simulink library "powerlib_modelsV2"  (Simulink 6.0)
settings: Solver=ode45  SolverMode=SingleTasking  StartTime=0.0  StopTime=10.0  RelTol=1e-3
undefined symbols (not defined in the file or in its folder): A, Ac, B, Bc, C, Cc, Cs, Current, damp, Dc, Dd, DiscIntNeverNeededParam, dref, dwo, exc, F, fb, gate, GH, GHd, GI, GId, GL, GLd, H, HT, hyd, ib, ib2, io, isfinite, j, K, Kd, Kg, L, Lad, Laq, lim, LIM, Ll, Llfd, Llkd, Llkq1, Llkq2, Llr, Lls, LowerFlux, N, N2, Nb, Nb2, nb_arm, p, Par_HarmoA_pu, Par_HarmoB_pu, Par_Timing_Harmo, Par_Timing_Variation, Par_Vps, Pb ... (+58)
libraries: powerlib_extras x14
(part 6 of 11)

== system powerlib_modelsV2/Continuous/Dynamic_Load/Break  Alg. Loop ==
  In : Inport  Orientation=left  Port=1  LatchInput=off
  Complex to Real-Imag : ComplexToRealImag  Orientation=left
  Real-Imag to Complex : RealImagToComplex  Orientation=left
  imag : Subsystem  Orientation=left  AncestorBlock=|  mask(Transfer Function with Initial Outputs){N=[1], D=[100e-6  1], Y0=imag(I1_init*exp(-j*Pha_V0*pi/180)), U0=imag(I1_init*exp(-j*Pha_V0*pi/180))}
      | simulink_extras/Additional
      | Linear/Transfer Fcn
      | (with initial outputs)
      mask prompts: N "Numerator:"; D "Denominator:"; Y0 "Initial output:"; U0 "Initial input:"
      mask help: Vector expressions for numerator, and denominator. Coefficients are in descending powers of s.
      mask init:
      | [A,B,C,Dd]=tf2ss(N,D);if (isempty(Y0));[m,n]=size(A);X0=zeros(1,m); end; if (isempty(U0));[m,p]=size(B);U0=zeros(1,p);end;X0=getxo(A,B,C,Dd,U0,Y0,0);
      mask Help: Specify the initial output for the transfer function.  An optimization routine attempts to determine the appropriate initial states so that the specified initial output is achieved.  For more details, see the m-file getxo.m
      mask Display: dpoly(N,D,'s')
  real : Subsystem  Orientation=left  AncestorBlock=|  mask(Transfer Function with Initial Outputs){N=[1], D=[100e-6  1], Y0=real(I1_init*exp(-j*Pha_V0*pi/180)), U0=real(I1_init*exp(-j*Pha_V0*pi/180))}
      | simulink_extras/Additional
      | Linear/Transfer Fcn
      | (with initial outputs)
      mask prompts: N "Numerator:"; D "Denominator:"; Y0 "Initial output:"; U0 "Initial input:"
      mask help: Vector expressions for numerator, and denominator. Coefficients are in descending powers of s.
      mask init:
      | [A,B,C,Dd]=tf2ss(N,D);if (isempty(Y0));[m,n]=size(A);X0=zeros(1,m); end; if (isempty(U0));[m,p]=size(B);U0=zeros(1,p);end;X0=getxo(A,B,C,Dd,U0,Y0,0);
      mask Help: Specify the initial output for the transfer function.  An optimization routine attempts to determine the appropriate initial states so that the specified initial output is achieved.  For more details, see the m-file getxo.m
      mask Display: dpoly(N,D,'s')
  Out : Outport  Orientation=left
  wires:
  In/1 -> Complex to Real-Imag/1
  Real-Imag to Complex/1 -> Out/1
  Complex to Real-Imag/1 -> real/1(In1)
  real/1(Out1) -> Real-Imag to Complex/1
  Complex to Real-Imag/2 -> imag/1(In1)
  imag/1(Out1) -> Real-Imag to Complex/2

== system powerlib_modelsV2/Continuous/Dynamic_Load/Positive Sequence  current ==
  note: I1= (S/V1)'
  note: V>Vmin :
      |
      |    P=Po*(V/Vo)^np
      |    Q=Qo*(V/Vo)^np
  note: V<Vmin
      | Constant impedance load :
      |
      |  P=Po*kp*V^2
      | Q=Qo*kq*V^2
  note: kp=Vmin^(np-2)/Vo^np
      | kq=Vmin^(nq-2)/Vo^nq
  V1(pu) : Inport  Port=1  LatchInput=off
  S_ext : Inport  Port=2  LatchInput=off
  Complex to Magnitude-Angle : ComplexToMagnitudeAngle  Output=Magnitude
  Complex to Real-Imag1 : ComplexToRealImag
  Conj1 : Math  Operator=conj  SaturateOnIntegerOverflow=on
  Math Function : Math  Operator=square  SaturateOnIntegerOverflow=on
  Mux1 : Mux  Inputs=3
  Mux2 : Mux  Inputs=2
  Mux3 : Mux  Inputs=2
  P0/ (Vo^np) : Gain  Gain=P0/(Mag_V0^np)  SaturateOnIntegerOverflow=on
  PQ_ext : Constant  Value=PQext
  Product : Product  Inputs=/*  SaturateOnIntegerOverflow=on  InputSameDT=on
  Q0/(Vo^nq) : Gain  Gain=Q0/(Mag_V0^nq)  SaturateOnIntegerOverflow=on
  Real-Imag to Complex : RealImagToComplex
  Switch1 : Switch  Threshold=0.5  InputSameDT=on
  Switch3 : Switch  Threshold=Vmin  InputSameDT=on
  Switch4 : Switch  Threshold=Vmin  InputSameDT=on
  TF_P : Subsystem  mask(Transfer function){T1=Tp1, T2=Tp2, V_Init=P0}
      mask prompts: T1 "Time constant T1 (s):"; T2 "Time constant T2 (s):"; V_Init "Initial input and output :"
      mask help:
      | This block implements a continuous transfer function:
      |
      |          1+T1s
      | H(s)= ------
      |          1+T2s
      |
      | States are initialized according to  initial input and output value so that simulation starts in steady state.
      mask init:
      | numc=[T1 1];
      | denc=[T2 1];
      | [Ac,Bc,Cc,Dc]=tf2ss(numc,denc);
      | 
      | % Compute Initial states
      | I=eye(size(Ac));
      | x0c=inv(-Ac)*Bc*V_Init;
      mask Display: disp('1+T1s\n---\n1+T2s')
  TF_Q : Subsystem  mask(Transfer function){T1=Tq1, T2=Tq2, V_Init=Q0}
      mask prompts: T1 "Time constant T1 (s):"; T2 "Time constant T2 (s):"; V_Init "Initial input and output :"
      mask help:
      | This block implements a continuous transfer function:
      |
      |          1+T1s
      | H(s)= ------
      |          1+T2s
      |
      | States are initialized according to  initial input and output value so that simulation starts in steady state.
      mask init:
      | numc=[T1 1];
      | denc=[T2 1];
      | [Ac,Bc,Cc,Dc]=tf2ss(numc,denc);
      | 
      | % Compute Initial states
      | I=eye(size(Ac));
      | x0c=inv(-Ac)*Bc*V_Init;
      mask Display: disp('1+T1s\n---\n1+T2s')
  V^nq : Fcn  Expr=u[1]^u[2]
  V^nq , : Fcn  Expr=u[1]^u[2]
  Vmin^(np-2) : Gain  Gain=Vmin^(np-2)  SaturateOnIntegerOverflow=on
  Vmin^(nq-2) : Gain  Gain=Vmin^(nq-2)  SaturateOnIntegerOverflow=on
  np : Constant  Value=np
  nq : Constant  Value=nq
  pu>V : Gain  Gain=Vnom*sqrt(3)/sqrt(2)  SaturateOnIntegerOverflow=on
  I1(A) : Outport
  VPQ : Outport  Port=2
  wires:
  TF_Q/1(Out1) -> Real-Imag to Complex/2
  TF_P/1(Out1) -> Real-Imag to Complex/1
  Complex to Real-Imag1/2 -> Mux1/3
  Complex to Real-Imag1/1 -> Mux1/2
  Mux1/1 -> VPQ/1
  Complex to Magnitude-Angle/1 -> Mux1/1, Switch4/2, Switch3/2, Mux2/1, Mux3/1, Math Function/1
  pu>V/1 -> Product/1
  PQ_ext/1 -> Switch1/2
  S_ext/1 -> Switch1/1
  Real-Imag to Complex/1 -> Switch1/3  "S_dyn"
  Switch1/1 -> Complex to Real-Imag1/1, Product/2  "S=P+jQ"
  Conj1/1 -> I1(A)/1
  Product/1 -> Conj1/1
  Switch4/1 -> Q0/(Vo^nq)/1
  P0/ (Vo^np)/1 -> TF_P/1(In1)
  Q0/(Vo^nq)/1 -> TF_Q/1(In1)
  Switch3/1 -> P0/ (Vo^np)/1
  np/1 -> Mux2/2
  Mux2/1 -> V^nq ,/1
  nq/1 -> Mux3/2
  Mux3/1 -> V^nq/1
  V1(pu)/1 -> pu>V/1, Complex to Magnitude-Angle/1
  V^nq/1 -> Switch4/1
  Math Function/1 -> Vmin^(np-2)/1, Vmin^(nq-2)/1
  Vmin^(np-2)/1 -> Switch3/3
  V^nq ,/1 -> Switch3/1
  Vmin^(nq-2)/1 -> Switch4/3

== system powerlib_modelsV2/Continuous/Dynamic_Load/Variable Frequency Mean value1 ==
  note: Pierre Giroux, Gilbert Sybille
      | Power System Simulation Laboratory
      | IREQ, Hydro-Quebc
  note: Mean Value (Variable frequency)
  Freq : Inport  Port=1  LatchInput=off
  In : Inport  Port=2  LatchInput=off
  Constant : Constant  Value=Vinit
  Integrator : Integrator
  Number of samples per cycle : Fcn  Expr=1/u[1]
  Product : Product  SaturateOnIntegerOverflow=on  InputSameDT=on
  Step : Step  Time=1/Finit  SampleTime=0
  Sum7 : Sum  Inputs=-+  SaturateOnIntegerOverflow=on  InputSameDT=on
  Switch : Switch  Threshold=0.5  InputSameDT=on
  To avoid division by zero : Saturate  Orientation=down  UpperLimit=1e6  LowerLimit=1e-6
  Variable Transport Delay : VariableTransportDelay  MaximumDelay=1/40  MaximumPoints=4096
  Mean : Outport
  wires:
  In/1 -> Integrator/1  "In"
  Product/1 -> Switch/1  "Mean value"
  Variable Transport Delay/1 -> Sum7/1
  Sum7/1 -> Product/1
  Integrator/1 -> Sum7/2, Variable Transport Delay/1
  Freq/1 -> Product/2, To avoid division by zero/1  "Freq"
  Constant/1 -> Switch/3
  Switch/1 -> Mean/1
  To avoid division by zero/1 -> Number of samples per cycle/1  "Freq"
  Step/1 -> Switch/2
  Number of samples per cycle/1 -> Variable Transport Delay/2  "Delay"

== system powerlib_modelsV2/Continuous/Dynamic_Load/Variable Frequency Mean value2 ==
  note: Mean Value (Variable frequency)
  note: Pierre Giroux, Gilbert Sybille
      | Power System Simulation Laboratory
      | IREQ, Hydro-Quebc
  Freq : Inport  Port=1  LatchInput=off
  In : Inport  Port=2  LatchInput=off
  Constant : Constant  Value=Vinit
  Integrator : Integrator
  Number of samples per cycle : Fcn  Expr=1/u[1]
  Product : Product  SaturateOnIntegerOverflow=on  InputSameDT=on
  Step : Step  Time=1/Finit  SampleTime=0
  Sum7 : Sum  Inputs=-+  SaturateOnIntegerOverflow=on  InputSameDT=on
  Switch : Switch  Threshold=0.5  InputSameDT=on
  To avoid division by zero : Saturate  Orientation=down  UpperLimit=1e6  LowerLimit=1e-6
  Variable Transport Delay : VariableTransportDelay  MaximumDelay=1/40  MaximumPoints=4096
  Mean : Outport
  wires:
  Number of samples per cycle/1 -> Variable Transport Delay/2  "Delay"
  Step/1 -> Switch/2
  To avoid division by zero/1 -> Number of samples per cycle/1  "Freq"
  Switch/1 -> Mean/1
  Constant/1 -> Switch/3
  Freq/1 -> To avoid division by zero/1, Product/2  "Freq"
  Integrator/1 -> Variable Transport Delay/1, Sum7/2
  Sum7/1 -> Product/1
  Variable Transport Delay/1 -> Sum7/1
  Product/1 -> Switch/1  "Mean value"
  In/1 -> Integrator/1  "In"

== system powerlib_modelsV2/Continuous/Dynamic_Load/dq0_to_abc Transformation ==
  note: Va= Vd*sinwt + Vq*cos(wt) + Vo
  note: sin
  note: cos
  note: cos
  note: Vb= Vd*sin(wt-2pi/3) + Vq*cos(wt-2pi/3) + Vo
  note: Vc= Vd*sin(wt+2pi/3) + Vq*cos(wt+2pi/3) + Vo
  dq0 : Inport  Port=1  PortDimensions=3  LatchInput=off
  sin_cos : Inport  Port=2  PortDimensions=2  LatchInput=off
  Demux : Demux  Outputs=2
  Fcn2 : Fcn  Expr="u[1]*u[4] +  u[2]*u[5] + u[3]"
  Fcn4 : Fcn  Expr="u[1]*u[6] +  u[2]*u[7]+ u[3]"
  Fcn5 : Fcn  Expr="u[1]*u[8]+  u[2]*u[9]+ u[3]"
  K1 : Constant  Value=0.5
  K2 : Constant  Value=sqrt(3)/2
  Mux : Mux  Inputs=2
  Mux1 : Mux  Inputs=3
  Mux2 : Mux  Inputs=6
  Product{,1..3} (4 alike) : Product  SaturateOnIntegerOverflow=on  InputSameDT=on
  Sum : Sum  Inputs=--  SaturateOnIntegerOverflow=on  InputSameDT=on
  Sum1 : Sum  Inputs=-+  SaturateOnIntegerOverflow=on  InputSameDT=on
  Sum2 : Sum  Inputs=--  SaturateOnIntegerOverflow=on  InputSameDT=on
  Sum3 : Sum  Inputs=--  SaturateOnIntegerOverflow=on  InputSameDT=on
  abc : Outport  InitialOutput=0
  wires:
  Fcn5/1 -> Mux1/3  "Vc"
  Fcn2/1 -> Mux1/1  "Va"
  Mux1/1 -> abc/1
  Mux/1 -> Fcn4/1, Fcn2/1, Fcn5/1
  Sum1/1 -> Sum3/1, Mux2/4  "cos(wt-2pi/3)"
  Sum/1 -> Sum2/1, Mux2/3  "sin(wt-2pi/3)"
  K2/1 -> Product2/2, Product1/2
  K1/1 -> Product3/2, Product/2
  Sum2/1 -> Mux2/5  "sin(wt+2pi/3)"
  Sum3/1 -> Mux2/6  "cos(wt+2pi/3)"
  Product2/1 -> Sum1/2
  Product3/1 -> Sum1/1
  Product1/1 -> Sum/2
  Product/1 -> Sum/1
  Demux/1 -> Mux2/1, Sum2/2, Product2/1, Product/1  "sin(wt)"
  Demux/2 -> Mux2/2, Product1/1, Product3/1, Sum3/2  "cos(wt)"
  sin_cos/1 -> Demux/1
  Mux2/1 -> Mux/2
  dq0/1 -> Mux/1  "Vabc"
  Fcn4/1 -> Mux1/2  "Vb"

== system powerlib_modelsV2/Continuous/Excitation_System/Damping kf.s\ (tf.s +1) ==
  In1 : Inport  Port=1  LatchInput=off
  State Space : StateSpace  A=A  B=B  C=C  D=Dd  X0=X0
  Out1 : Outport  InitialOutput=0
  wires:
  State Space/1 -> Out1/1
  In1/1 -> State Space/1

== system powerlib_modelsV2/Continuous/Excitation_System/Exciter 1 \(te.s +ke) ==
  In1 : Inport  Port=1  LatchInput=off
  State Space : StateSpace  A=A  B=B  C=C  D=Dd  X0=X0
  Out1 : Outport  InitialOutput=0
  wires:
  In1/1 -> State Space/1
  State Space/1 -> Out1/1

== system powerlib_modelsV2/Continuous/Excitation_System/Lead Lag Compensator tc.s+1\tb.s+1 ==
  In1 : Inport  Port=1  LatchInput=off
  State Space : StateSpace  A=A  B=B  C=C  D=Dd  X0=X0
  Out1 : Outport  InitialOutput=0
  wires:
  State Space/1 -> Out1/1
  In1/1 -> State Space/1

== system powerlib_modelsV2/Continuous/Excitation_System/Low Pass Filter 1 \ (tr.s+1) (with IC) ==
  In1 : Inport  Port=1  LatchInput=off
  State Space : StateSpace  A=A  B=B  C=C  D=Dd  X0=X0
  Out1 : Outport  InitialOutput=0
  wires:
  In1/1 -> State Space/1
  State Space/1 -> Out1/1

== system powerlib_modelsV2/Continuous/Excitation_System/Main Regulator ka \ (ta.s+1) ==
  In1 : Inport  Port=1  LatchInput=off
  State Space : StateSpace  A=A  B=B  C=C  D=Dd  X0=X0
  Out1 : Outport  InitialOutput=0
  wires:
  State Space/1 -> Out1/1
  In1/1 -> State Space/1

== system powerlib_modelsV2/Continuous/Excitation_System/proportionnal saturation ==
  Efd : Inport  Port=1  LatchInput=off
  Vtf : Inport  Port=2  LatchInput=off
  Constant : Constant  Value=kp
  Constant1 : Constant  Value=efmin
  Constant3 : Constant  Value=0
  Data Type  Conversion{,1..3} (4 alike) : DataTypeConversion  SaturateOnIntegerOverflow=on  RndMeth=Zero
  Logical Operator : Logic
  Logical Operator1 : Logic  Operator=NOT  Inputs=1
  Logical Operator2 : Logic  Operator=NOT  Inputs=1
  Product : Product  SaturateOnIntegerOverflow=on  InputSameDT=on
  Product1 : Product  SaturateOnIntegerOverflow=on  InputSameDT=on
  Product2 : Product  SaturateOnIntegerOverflow=on  InputSameDT=on
  Relational Operator : RelationalOperator  Operator===  InputSameDT=on
  Relational Operator1 : RelationalOperator  Operator=<  InputSameDT=on
  Relational Operator2 : RelationalOperator  Operator=>  InputSameDT=on
  Sum : Sum  SaturateOnIntegerOverflow=on  InputSameDT=on
  Sum1 : Sum  Inputs=+++  SaturateOnIntegerOverflow=on  InputSameDT=on
  Vfdmax : Gain  Gain=efmax  SaturateOnIntegerOverflow=on
  Vfdmax1 : Gain  Gain=kp  SaturateOnIntegerOverflow=on
  Ef : Outport  InitialOutput=0
  wires:
  Data Type  Conversion3/1 -> Vfdmax/1
  Relational Operator/1 -> Data Type  Conversion3/1
  Data Type  Conversion2/1 -> Product2/1
  Logical Operator2/1 -> Data Type  Conversion2/1
  Data Type  Conversion1/1 -> Product1/2
  Logical Operator1/1 -> Data Type  Conversion1/1
  Data Type  Conversion/1 -> Product/2
  Logical Operator/1 -> Data Type  Conversion/1
  Product1/1 -> Sum1/2
  Product2/1 -> Sum1/3
  Product/1 -> Sum1/1
  Sum1/1 -> Ef/1
  Efd/1 -> Product/1, Relational Operator1/1, Relational Operator2/1
  Constant1/1 -> Product1/1, Relational Operator2/2
  Relational Operator1/1 -> Logical Operator/2, Logical Operator2/1
  Relational Operator2/1 -> Logical Operator/1, Logical Operator1/1
  Sum/1 -> Relational Operator1/2, Product2/2
  Vfdmax1/1 -> Sum/1
  Vfdmax/1 -> Sum/2
  Constant3/1 -> Relational Operator/2
  Constant/1 -> Relational Operator/1
  Vtf/1 -> Vfdmax1/1

== system powerlib_modelsV2/Continuous/GTO-IGBT Bridge/Diode Logic ==
  note: Note : Block D1 (D2) if D2 (D1) is triggered (no Cs)
  Vak : Inport  Port=1  LatchInput=off
  Ipos : Inport  Port=2  LatchInput=off
  G : Inport  Port=3  LatchInput=off
  0 2 : Constant  Value=0
  0 3 : Constant  Value=Cs==inf
  1 : Logic
  2 : Logic  Operator=OR
  3 : Logic  Operator=OR
  Block D : Selector  Orientation=up  Elements=Selec_Diode  InputPortWidth=nb_switch
  Blocking Diodes : Subsystem
  Data Type  Conversion3 : DataTypeConversion  SaturateOnIntegerOverflow=on  RndMeth=Zero
  Logical Operator3 : Logic  Operator=NOT
  Trig.  Diodes (No Snubber Capacitance) : Subsystem  TreatAsAtomicUnit=on
  b6 : RelationalOperator  Operator=>  InputSameDT=on
  status : Outport  InitialOutput=0
  wires:
  0 3/1 -> Trig.  Diodes (No Snubber Capacitance)/Enable
  Ipos/1 -> Trig.  Diodes (No Snubber Capacitance)/2(Ipos)
  G/1 -> Trig.  Diodes (No Snubber Capacitance)/1(G), Blocking Diodes/1(G)
  0 2/1 -> b6/2
  Vak/1 -> b6/1
  Blocking Diodes/1(Block.D) -> 3/1
  2/1 -> status/1
  1/1 -> 2/1
  Logical Operator3/1 -> 1/2
  3/1 -> Logical Operator3/1
  Trig.  Diodes (No Snubber Capacitance)/1(Trig D) -> 2/2, Block D/1
  Block D/1 -> 3/2
  b6/1 -> Data Type  Conversion3/1
  Data Type  Conversion3/1 -> 1/1

== system powerlib_modelsV2/Continuous/GTO-IGBT Bridge/GTO Logic ==
  Vak : Inport  Port=1  LatchInput=off
  G : Inport  Port=2  LatchInput=off
  " " : RelationalOperator  Operator=>  InputSameDT=on
  "    " : Constant  Value=0
  ". " : Logic
  Data Type  Conversion1 : DataTypeConversion  SaturateOnIntegerOverflow=on  RndMeth=Zero
  Data Type  Conversion3 : DataTypeConversion  SaturateOnIntegerOverflow=on  RndMeth=Zero
  Data Type  Conversion4 : DataTypeConversion  SaturateOnIntegerOverflow=on  RndMeth=Zero
  Vpos : Constant  Value=0
  b : RelationalOperator  Operator=>  InputSameDT=on
  status : Outport  InitialOutput=0
  wires:
  ". "/1 -> status/1
  Vak/1 -> b/1
  Vpos/1 -> b/2
  G/1 -> " "/1
  b/1 -> Data Type  Conversion1/1
  Data Type  Conversion1/1 -> ". "/1
  " "/1 -> Data Type  Conversion3/1
  Data Type  Conversion3/1 -> ". "/2
  "    "/1 -> Data Type  Conversion4/1
  Data Type  Conversion4/1 -> " "/2

== system powerlib_modelsV2/Continuous/GTO-IGBT Bridge/Tail  ==
  Iak : Inport  Port=1  LatchInput=off
  switch : Inport  Port=2  LatchInput=off
  Enable : EnablePort  StatesWhenEnabling=reset
  1 : Constant
  2 : Constant  Value=(Tf+Tt)>0
  Data Type  Conversion1 : DataTypeConversion  SaturateOnIntegerOverflow=on  RndMeth=Zero
  Integrator : Integrator  ExternalReset=falling
  Look-Up Table : Lookup  DialogController=Simulink.DDGSource  InputValues="[  0   Tf+eps Tf+Tt+2*eps  Tf+Tt+3*eps]"  OutputValues="[  1   0.1*(Tt>0) 0 0]"  SaturateOnIntegerOverflow=on
  Memory : Memory  Orientation=left  InheritSampleTime=on
  Product : Product  Inputs=3  SaturateOnIntegerOverflow=on  InputSameDT=on
  Switch : Switch  Threshold=0.5  InputSameDT=on
  itail : Outport  InitialOutput=0
  wires:
  2/1 -> Data Type  Conversion1/1
  Look-Up Table/1 -> Product/1
  1/1 -> Integrator/1
  Iak/1 -> Switch/1
  switch/1 -> Switch/2, Integrator/2
  Integrator/1 -> Look-Up Table/1
  Product/1 -> itail/1
  Switch/1 -> Product/2, Memory/1
  Memory/1 -> Switch/3
  Data Type  Conversion1/1 -> Product/3

== system powerlib_modelsV2/Continuous/GTO-IGBT Bridge/Vf  ==
  status_GTO : Inport  Port=1  LatchInput=off
  Switch : Switch  Threshold=0.5  InputSameDT=on
  Vf device : Constant  Value=Vf*ones(nb_switch,1)
  Vf diode : Constant  Value=-Vfd*ones(nb_switch,1)
  Vf : Outport  InitialOutput=[0]
  wires:
  status_GTO/1 -> Switch/2
  Switch/1 -> Vf/1
  Vf diode/1 -> Switch/3
  Vf device/1 -> Switch/1

== system powerlib_modelsV2/Continuous/HTG/PID ==
  error : Inport  Port=1  LatchInput=off
  Derivative : TransferFcn  Numerator=[ kd 0]  Denominator=[ td 1 ]
  Integral : Gain  Gain=ki  SaturateOnIntegerOverflow=on
  Integrator1 : Integrator  InitialCondition=go
  Proportional : Gain  Gain=kp  SaturateOnIntegerOverflow=on
  Sum : Sum  Inputs=+++  SaturateOnIntegerOverflow=on  InputSameDT=on
  Output : Outport  InitialOutput=0
  wires:
  Integrator1/1 -> Sum/2
  Integral/1 -> Integrator1/1
  error/1 -> Integral/1, Proportional/1, Derivative/1
  Sum/1 -> Output/1
  Derivative/1 -> Sum/3
  Proportional/1 -> Sum/1

== system powerlib_modelsV2/Continuous/HTG/servo-motor ==
  regulator's output : Inport  Port=1  LatchInput=off
  Sum4 : Sum  Inputs=+-  SaturateOnIntegerOverflow=on  InputSameDT=on
  position : Integrator  InitialCondition=go  LimitOutput=on  UpperSaturationLimit=gmax  LowerSaturationLimit=gmin
  servo- motor : TransferFcn  Numerator=[ka]  Denominator=[ta 1]
  speed limit : Saturate  UpperLimit=vgmax  LowerLimit=vgmin
  gate opening : Outport  InitialOutput=0
  wires:
  position/1 -> Sum4/2, gate opening/1
  speed limit/1 -> position/1
  servo- motor/1 -> speed limit/1
  Sum4/1 -> servo- motor/1
  regulator's output/1 -> Sum4/1

== system powerlib_modelsV2/Continuous/HTG/turbine ==
  dw : Inport  Port=1  LatchInput=off
  gate opening : Inport  Port=2  LatchInput=off
  Constant : Constant  Orientation=left
  Fcn : Fcn  Expr=(u(2)/u(1))^2
  Gain2 : Gain  Orientation=left  Gain=1/tw  SaturateOnIntegerOverflow=on
  Integrator : Integrator  Orientation=left  InitialCondition=po
  Mux : Mux  Inputs=2
  Product : Product  SaturateOnIntegerOverflow=on  InputSameDT=on
  Sum2 : Sum  Inputs=-+  SaturateOnIntegerOverflow=on  InputSameDT=on
  Sum3 : Sum  Orientation=left  Inputs=-+  SaturateOnIntegerOverflow=on  InputSameDT=on
  beta : Gain  Gain=beta  SaturateOnIntegerOverflow=on
  turbine gain : Gain  Gain=1/(gmax-gmin)  SaturateOnIntegerOverflow=on
  Pm : Outport  InitialOutput=0
  wires:
  turbine gain/1 -> Mux/1
  gate opening/1 -> turbine gain/1
  Integrator/1 -> Product/2, Mux/2
  Mux/1 -> Fcn/1
  Fcn/1 -> Sum2/2
  Constant/1 -> Sum3/2
  Product/1 -> Pm/1
  Sum3/1 -> Gain2/1
  Gain2/1 -> Integrator/1
  Sum2/1 -> Sum3/1, Product/1
  beta/1 -> Sum2/1
  dw/1 -> beta/1

== system powerlib_modelsV2/Continuous/MBPSS/Transfer function for detailed model (HF) ==
  On : Inport  Port=1  LatchInput=off
  "HFpos " : Inport  Port=2  LatchInput=off
  "HFneg " : Inport  Port=3  LatchInput=off
  Switch1 : Switch  Threshold=0.5  InputSameDT=on
  Switch2 : Switch  Threshold=0.5  InputSameDT=on
  Transfer functions for detailed stabilizer : Subsystem  TreatAsAtomicUnit=on
  Transfer functions for detailed stabilizer2 : Subsystem  TreatAsAtomicUnit=on
  HFpos : Outport
  HFneg : Outport  Port=2
  wires:
  Transfer functions for detailed stabilizer/1(Out1) -> Switch1/1
  "HFpos "/1 -> Transfer functions for detailed stabilizer/1(In1), Switch1/3
  Switch1/1 -> HFpos/1
  "HFneg "/1 -> Transfer functions for detailed stabilizer2/1(In1), Switch2/3
  Switch2/1 -> HFneg/1
  Transfer functions for detailed stabilizer2/1(Out1) -> Switch2/1
  On/1 -> Transfer functions for detailed stabilizer/Enable, Switch1/2, Switch2/2, Transfer functions for detailed stabilizer2/Enable

== system powerlib_modelsV2/Continuous/MBPSS/Transfer function for detailed model (IF) ==
  On : Inport  Port=1  LatchInput=off
  "IFpos " : Inport  Port=2  LatchInput=off
  "IFneg " : Inport  Port=3  LatchInput=off
  Switch1 : Switch  Threshold=0.5  InputSameDT=on
  Switch2 : Switch  Threshold=0.5  InputSameDT=on
  Transfer functions for detailed stabilizer : Subsystem  TreatAsAtomicUnit=on
  Transfer functions for detailed stabilizer2 : Subsystem  TreatAsAtomicUnit=on
  IFpos : Outport
  LFneg : Outport  Port=2
  wires:
  On/1 -> Transfer functions for detailed stabilizer2/Enable, Switch2/2, Switch1/2, Transfer functions for detailed stabilizer/Enable
  Transfer functions for detailed stabilizer2/1(Out1) -> Switch2/1
  Switch2/1 -> LFneg/1
  "IFneg "/1 -> Switch2/3, Transfer functions for detailed stabilizer2/1(In1)
  Switch1/1 -> IFpos/1
  "IFpos "/1 -> Switch1/3, Transfer functions for detailed stabilizer/1(In1)
  Transfer functions for detailed stabilizer/1(Out1) -> Switch1/1

== system powerlib_modelsV2/Continuous/MBPSS/Transfer function for detailed model (LF) ==
  On : Inport  Port=1  LatchInput=off
  "LFpos " : Inport  Port=2  LatchInput=off
  "LFneg " : Inport  Port=3  LatchInput=off
  Switch1 : Switch  Threshold=0.5  InputSameDT=on
  Switch2 : Switch  Threshold=0.5  InputSameDT=on
  Transfer functions for detailed stabilizer : Subsystem  TreatAsAtomicUnit=on
  Transfer functions for detailed stabilizer2 : Subsystem  TreatAsAtomicUnit=on
  LFpos : Outport
  LFneg : Outport  Port=2
  wires:
  Transfer functions for detailed stabilizer/1(Out1) -> Switch1/1
  "LFpos "/1 -> Transfer functions for detailed stabilizer/1(In1), Switch1/3
  Switch1/1 -> LFpos/1
  "LFneg "/1 -> Transfer functions for detailed stabilizer2/1(In1), Switch2/3
  Switch2/1 -> LFneg/1
  Transfer functions for detailed stabilizer2/1(Out1) -> Switch2/1
  On/1 -> Transfer functions for detailed stabilizer/Enable, Switch1/2, Switch2/2, Transfer functions for detailed stabilizer2/Enable

== system powerlib_modelsV2/Continuous/PM_synchronous_machine/abc2qd ==
  note: This subsystem converts Vab and Vbc to Vd,Vq. The sine and cosine com-
      | puted here are sent to the inverse transformation subsystem dq2abc.
  Vab,Vbc : Inport  Port=1  LatchInput=off
  the : Inport  Port=2  LatchInput=off
  Elementary Math : ElementaryMath
  Elementary Math1 : ElementaryMath  Operator=cos
  Fcn2 : Fcn  Expr=(u[4]*(2*u[1]+u[2]) + (sqrt3*u[2]*u[3])) * one_third
  Fcn3 : Fcn  Expr=(u[3]*(2*u[1]+u[2]) + (-sqrt3*u[2]*u[4])) * one_third
  Mux1 : Mux  Inputs=[ 2 2 ]
  Mux2 : Mux  Inputs=2
  Mux3 : Mux  Inputs=2
  s,c : Outport  InitialOutput=0
  vq,vd : Outport  Port=2  InitialOutput=0
  wires:
  the/1 -> Elementary Math1/1, Elementary Math/1
  Elementary Math1/1 -> Mux3/2
  Elementary Math/1 -> Mux3/1
  Vab,Vbc/1 -> Mux1/1
  Mux2/1 -> vq,vd/1
  Fcn3/1 -> Mux2/2
  Fcn2/1 -> Mux2/1
  Mux3/1 -> Mux1/2, s,c/1
  Mux1/1 -> Fcn3/1, Fcn2/1

== system powerlib_modelsV2/Continuous/PM_synchronous_machine/iq,id ==
  vq,vd : Inport  Port=1  LatchInput=off
  we : Inport  Port=2  LatchInput=off
  Demux : Demux  Outputs=2
  Mux : Mux  Inputs=2
  id : Subsystem
  iq : Subsystem
  iq,id : Outport  InitialOutput=0
  wires:
  Mux/1 -> iq,id/1
  vq,vd/1 -> Demux/1
  Demux/1 -> iq/1(vq)
  Demux/2 -> id/3(vd)
  iq/1(iq) -> id/1(iq), Mux/1
  id/1(id) -> iq/3(id), Mux/2
  we/1 -> id/2(we), iq/2(we)

== system powerlib_modelsV2/Continuous/PM_synchronous_machine/mec ==
  Tm : Inport  Port=1  LatchInput=off
  iq,id : Inport  Port=2  LatchInput=off
  Gain : Gain  Gain=p  SaturateOnIntegerOverflow=on
  Gain1 : Gain  Gain=1/p  SaturateOnIntegerOverflow=on
  Gain2 : Gain  Gain=1/J  SaturateOnIntegerOverflow=on
  Gain3 : Gain  Gain=F  SaturateOnIntegerOverflow=on
  Int : Integrator
  Int1 : Integrator
  Mux1 : Mux  Inputs=3
  Sum : Sum  Inputs=-+-  SaturateOnIntegerOverflow=on  InputSameDT=on
  Te : Fcn  Expr=1.5*p*(lam*u(1)+(Ld-Lq)*u(1)*u(2))
  we : Outport  InitialOutput=0
  the : Outport  Port=2  InitialOutput=0
  w,th,Te : Outport  Port=3  InitialOutput=0
  wires:
  Gain3/1 -> Sum/3
  Mux1/1 -> w,th,Te/1
  Te/1 -> Sum/2, Mux1/3
  Tm/1 -> Sum/1
  Sum/1 -> Gain2/1
  Gain2/1 -> Int/1
  Int/1 -> Gain/1, Gain3/1, Mux1/1
  Gain/1 -> Int1/1, we/1
  iq,id/1 -> Te/1
  Gain1/1 -> Mux1/2
  Int1/1 -> the/1, Gain1/1

== system powerlib_modelsV2/Continuous/PM_synchronous_machine/qd2abc ==
  s,c : Inport  Port=1  LatchInput=off
  iq,id : Inport  Port=2  LatchInput=off
  Fcn : Fcn  Expr=u[3]*u[2] + u[4]*u[1]
  Fcn1 : Fcn  Expr=(u[2]*(-u[3]-sqrt3*u[4]) + u[1]*(sqrt3*u[3]-u[4]))*0.5
  Mux : Mux  Inputs=[2,2]
  Mux2 : Mux  Inputs=3
  Sum : Sum  Orientation=down  Inputs=--  SaturateOnIntegerOverflow=on  InputSameDT=on
  is : Outport  InitialOutput=0
  wires:
  Mux2/1 -> is/1
  Fcn1/1 -> Sum/1, Mux2/2
  Fcn/1 -> Sum/2, Mux2/1
  Sum/1 -> Mux2/3
  iq,id/1 -> Mux/2
  s,c/1 -> Mux/1
  Mux/1 -> Fcn1/1, Fcn/1

== system powerlib_modelsV2/Continuous/PSS/Sensor ==
  In : Inport  Port=1  LatchInput=off
  State-Space : StateSpace  A=Ac  B=Bc  C=Cc  D=Dc  X0=x0c
  Out : Outport  InitialOutput=0
  wires:
  In/1 -> State-Space/1
  State-Space/1 -> Out/1

== system powerlib_modelsV2/Continuous/PSS/Wash-out ==
  In : Inport  Port=1  LatchInput=off
  State-Space : StateSpace  A=Ac  B=Bc  C=Cc  D=Dc  X0=x0c
  Out : Outport  InitialOutput=0
  wires:
  In/1 -> State-Space/1
  State-Space/1 -> Out/1

== system powerlib_modelsV2/Continuous/Three-Level Bridge/2-level GTO-IGBT Bridge  Logic (modified) ==
  note: Diode Logic :
      | 1) Diodes are blocked when complementary GTOs are switched on
  note: Note 3: See Sw3 logic
  v : Inport  Port=1  LatchInput=off
  g : Inport  Port=2  LatchInput=off
  Block12 : Inport  Port=3  LatchInput=off
  Trig12 : Inport  Port=4  LatchInput=off
  Data Type  Conversion2 : DataTypeConversion  SaturateOnIntegerOverflow=on  RndMeth=Zero
  Data Type  Conversion4 : DataTypeConversion  SaturateOnIntegerOverflow=on  RndMeth=Zero
  Demux1 : Demux  Outputs=[nb_arm nb_arm]
  Diode Logic : Subsystem
  GTO Logic : Subsystem
  G_D : Logic  Operator=OR
  G_D2 : Logic  Operator=NOT
  G_D3 : Logic  Operator=OR
  G_D4 : Logic  Operator=OR
  Gain : Gain  Orientation=up  Gain=-1  SaturateOnIntegerOverflow=on
  Gain1 : Gain  Gain=2  SaturateOnIntegerOverflow=on
  Memory : Memory
  Memory1 : Memory
  Note 3 : Logic
  Select_Block3 : Selector  Elements=Block3Elements  InputPortWidth=nb_switch
  Select_Vsw : Selector  Elements=VswElements  InputPortWidth=nb_arm*3
  "Vf " : Subsystem
  status : Outport
  Vf : Outport  Port=2
  Block3 : Outport  Port=3
  status_GTO : Outport  Port=4
  wires:
  Demux1/2 -> G_D3/2
  Demux1/1 -> G_D3/1
  Select_Block3/1 -> Demux1/1
  Select_Vsw/1 -> GTO Logic/1(Vak), Gain/1
  Trig12/1 -> G_D4/2
  Note 3/1 -> G_D4/1
  G_D4/1 -> G_D/1
  Memory/1 -> Vf/1
  Data Type  Conversion2/1 -> Memory1/1
  G_D/1 -> Data Type  Conversion2/1
  Memory1/1 -> status/1
  Data Type  Conversion4/1 -> GTO Logic/2(G)
  g/1 -> Data Type  Conversion4/1
  GTO Logic/1(status) -> status_GTO/1, "Vf "/1(status_GTO), Diode Logic/2(G), G_D/2
  "Vf "/1(Vf) -> Gain1/1
  v/1 -> Select_Vsw/1
  Gain/1 -> Diode Logic/1(Vak)
  Diode Logic/2(block) -> Select_Block3/1
  Diode Logic/1(status) -> Note 3/1
  Block12/1 -> G_D2/1
  G_D2/1 -> Note 3/2
  Gain1/1 -> Memory/1
  G_D3/1 -> Block3/1

== system powerlib_modelsV2/Continuous/Three-Level Bridge/Input ==
  note: This block is required when the "pulses" input is not connected
  In : Inport  Port=1  LatchInput=off
  Constant : Constant
  require : Logic  OutDataTypeMode=Specify via dialog  LogicDataType=float('double')
  Out : Outport
  wires:
  require/1 -> Out/1
  In/1 -> require/1
  Constant/1 -> require/2

== system powerlib_modelsV2/Continuous/Three-Level Bridge/SubSystem ==
  note: (or B or C)
  note: (or B or C)
  note: <======>
  note: |
      | |
      | |
      | |
      | |
      | [Sw2]
      | |
      | |
      | |
      | |
  note: |
      | |
      | |
      | |
      | |
      | [Sw1]
      | |
      | |
      | |
      | |
  note: + Vdc ------------
  note: ---------- A
  note: + Vdc --------------------------
  note: - Vdc--------------------------
  note: N ----------
  note: |
      | |
      | |
      | |
      | |
      | |
      | |
      | |
      | |
      | |
      | |
  note: ------------ A
  note: -----<-[D6]---------
  note: -------[D5]-->-------
  note: |
      | |
      | [Q4 - D4]
      | |
      | |
      | |
  note: |
      | |
      | [Q3 - D3]
      | |
      | |
  note: |
      | |
      | [Q2 - D2]
      | |
      | |
  note: |
      | |
      | |
      | [Q1 - D1]
      | |
      | |
  note: -[Sw3]-----
  note: N ----
  note: - Vdc ------------
  note: D5, D6 : Clamping diodes

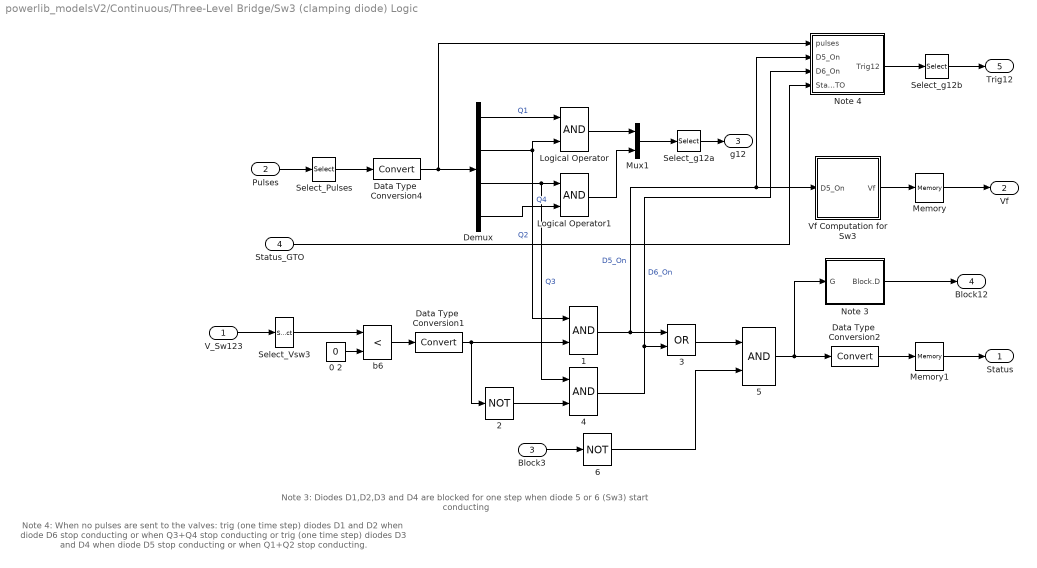
== system powerlib_modelsV2/Continuous/Three-Level Bridge/Sw3 (clamping diode) Logic ==
  note: Note 4: When no pulses are sent to the valves:
      | trig (one time step) diodes D1 and D2 when diode D6 stop conducting or when Q3+Q4 stop conducting
      | or trig (one time step) diodes D3 and D4 when diode D5 stop conducting or when Q1+Q2 stop conducting.
  note: Note 3: Diodes D1,D2,D3 and D4 are blocked for one step when diode 5 or 6 (Sw3) start conducting
  V_Sw123 : Inport  Port=1  LatchInput=off
  Pulses : Inport  Port=2  LatchInput=off
  Block3 : Inport  Port=3  LatchInput=off
  Status_GTO : Inport  Port=4  LatchInput=off
  0 2 : Constant  Value=0
  1 : Logic
  2 : Logic  Operator=NOT
  3 : Logic  Operator=OR
  4 : Logic
  5 : Logic
  6 : Logic  Operator=NOT
  Data Type  Conversion1 : DataTypeConversion  SaturateOnIntegerOverflow=on  RndMeth=Zero
  Data Type  Conversion2 : DataTypeConversion  SaturateOnIntegerOverflow=on  RndMeth=Zero
  Data Type  Conversion4 : DataTypeConversion  SaturateOnIntegerOverflow=on  RndMeth=Zero
  Demux : Demux  Outputs=[nb_arm nb_arm nb_arm nb_arm]
  Logical Operator : Logic
  Logical Operator1 : Logic
  Memory : Memory
  Memory1 : Memory
  Mux1 : Mux  Inputs=[nb_arm nb_arm]
  Note 3 : Subsystem
  Note 4 : Subsystem
  Select_Pulses : Selector  Elements=PulseElements  InputPortWidth=nb_arm*4
  Select_Vsw3 : Selector  Elements=Vsw3Elements  InputPortWidth=nb_arm*3
  Select_g12a : Selector  Elements=g12Elements  InputPortWidth=nb_arm*2
  Select_g12b : Selector  Elements=g12Elements  InputPortWidth=nb_arm*2
  Vf Computation for Sw3 : Subsystem
  b6 : RelationalOperator  Operator=<  InputSameDT=on
  Status : Outport
  Vf : Outport  Port=2
  g12 : Outport  Port=3
  Block12 : Outport  Port=4
  Trig12 : Outport  Port=5
  wires:
  Status_GTO/1 -> Note 4/4(Status_GTO)
  Select_Pulses/1 -> Data Type  Conversion4/1
  Note 4/1(Trig12) -> Select_g12b/1
  Data Type  Conversion2/1 -> Memory1/1
  6/1 -> 5/2
  3/1 -> 5/1
  1/1 -> Note 4/2(D5_On), Vf Computation for Sw3/1(D5_On), 3/1  "D5_On"
  4/1 -> Note 4/3(D6_On), 3/2  "D6_On"
  Data Type  Conversion1/1 -> 2/1, 1/2
  b6/1 -> Data Type  Conversion1/1
  Logical Operator1/1 -> Mux1/2
  Demux/4 -> Logical Operator1/2  "Q4"
  Demux/3 -> Logical Operator1/1, 4/1  "Q3"
  Demux/2 -> 1/1, Logical Operator/2  "Q2"
  Demux/1 -> Logical Operator/1  "Q1"
  Data Type  Conversion4/1 -> Note 4/1(pulses), Demux/1
  Memory/1 -> Vf/1
  Vf Computation for Sw3/1(Vf) -> Memory/1
  Mux1/1 -> Select_g12a/1
  Pulses/1 -> Select_Pulses/1
  0 2/1 -> b6/2
  V_Sw123/1 -> Select_Vsw3/1
  2/1 -> 4/2
  Memory1/1 -> Status/1
  Block3/1 -> 6/1
  Note 3/1(Block.D) -> Block12/1
  5/1 -> Data Type  Conversion2/1, Note 3/1(G)
  Select_Vsw3/1 -> b6/1
  Logical Operator/1 -> Mux1/1
  Select_g12a/1 -> g12/1
  Select_g12b/1 -> Trig12/1

== system powerlib_modelsV2/Continuous/asynchronous_machine/Mechanical ==
  Tm : Inport  Port=1  LatchInput=off
  phis,is : Inport  Port=2  LatchInput=off
  1\p : Gain  Gain=1/p  SaturateOnIntegerOverflow=on
  1_2H : Gain  Gain=1/(2*H)  SaturateOnIntegerOverflow=on
  1_Tb2 : Gain  Gain=1/Tb2  SaturateOnIntegerOverflow=on
  F : Gain  Orientation=left  Gain=F  SaturateOnIntegerOverflow=on
  Integrator : Integrator  InitialCondition=wmo
  Integrator1 : Integrator  InitialCondition=tho
  Mux3 : Mux  Inputs=2
  Mux4 : Mux  Inputs=3
  Product1 : Product  Inputs=1  SaturateOnIntegerOverflow=on  InputSameDT=on
  Product2 : Product  Inputs=1  SaturateOnIntegerOverflow=on  InputSameDT=on
  Selector : Selector  Elements=[1 4]  InputPortWidth=4
  Selector1 : Selector  Elements=[2 3]  InputPortWidth=4
  Sum : Sum  Inputs=-+-  SaturateOnIntegerOverflow=on  InputSameDT=on
  Sum1 : Sum  Inputs=|-+  SaturateOnIntegerOverflow=on  InputSameDT=on
  web_psb : Gain  Gain=web_psb  SaturateOnIntegerOverflow=on
  w,Te,thr : Outport
  thr,wr : Outport  Port=2
  wires:
  Integrator1/1 -> Mux3/1, 1\p/1
  1\p/1 -> Mux4/3
  web_psb/1 -> Integrator1/1
  Sum1/1 -> Sum/2, Mux4/2
  1_Tb2/1 -> Sum/1
  F/1 -> Sum/3
  Integrator/1 -> web_psb/1, Mux4/1, Mux3/2, F/1
  1_2H/1 -> Integrator/1
  Sum/1 -> 1_2H/1
  Tm/1 -> 1_Tb2/1
  Mux3/1 -> thr,wr/1
  Mux4/1 -> w,Te,thr/1
  Product1/1 -> Sum1/1
  Product2/1 -> Sum1/2
  phis,is/1 -> Selector/1, Selector1/1
  Selector1/1 -> Product2/1
  Selector/1 -> Product1/1

== system powerlib_modelsV2/Continuous/asynchronous_machine/Mutual fluxes ==
  phiqr,phidr : Inport  Port=1  LatchInput=off
  phiqs,phids : Inport  Port=2  LatchInput=off
  1\Llr : Gain  Gain=1/Llr  SaturateOnIntegerOverflow=on
  1\Llr1 : Gain  Gain=Laq  SaturateOnIntegerOverflow=on
  1\Llr2 : Gain  Gain=Lad  SaturateOnIntegerOverflow=on
  1\Lls : Gain  Gain=1/Lls  SaturateOnIntegerOverflow=on
  Demux1 : Demux  Outputs=2
  Demux2 : Demux  Outputs=2
  Mux3 : Mux  Inputs=2
  Sum : Sum  Inputs=|++  SaturateOnIntegerOverflow=on  InputSameDT=on
  Sum1 : Sum  Inputs=++|  SaturateOnIntegerOverflow=on  InputSameDT=on
  phimq,phimd : Outport
  wires:
  Mux3/1 -> phimq,phimd/1
  1\Llr2/1 -> Mux3/2
  1\Llr1/1 -> Mux3/1
  Demux1/2 -> Sum1/1
  Demux2/2 -> Sum1/2
  Demux2/1 -> Sum/2
  1\Lls/1 -> Demux2/1
  Sum/1 -> 1\Llr1/1
  Demux1/1 -> Sum/1
  1\Llr/1 -> Demux1/1
  phiqr,phidr/1 -> 1\Llr/1
  phiqs,phids/1 -> 1\Lls/1
  Sum1/1 -> 1\Llr2/1

== system powerlib_modelsV2/Continuous/asynchronous_machine/Rotor ==
  vqr,vdr : Inport  Port=1  LatchInput=off
  w-wr : Inport  Port=2  LatchInput=off
  phimq,phimd : Inport  Port=3  LatchInput=off
  1\Llr : Gain  Gain=1/Llr  SaturateOnIntegerOverflow=on
  1\Llr1 : Gain  Gain=Rr  SaturateOnIntegerOverflow=on
  1\Llr2 : Gain  Gain=1/Llr  SaturateOnIntegerOverflow=on
  1\Llr3 : Gain  Gain=Rr  SaturateOnIntegerOverflow=on
  Demux : Demux  Outputs=2
  Demux1 : Demux  Outputs=2
  Mux2 : Mux  Inputs=2
  Mux3 : Mux  Inputs=2
  Product : Product  SaturateOnIntegerOverflow=on  InputSameDT=on
  Product1 : Product  Orientation=left  SaturateOnIntegerOverflow=on  InputSameDT=on
  Sum1 : Sum  Inputs=++-||  SaturateOnIntegerOverflow=on  InputSameDT=on
  Sum2 : Sum  Inputs=+--  SaturateOnIntegerOverflow=on  InputSameDT=on
  Sum3 : Sum  Inputs=+-|  SaturateOnIntegerOverflow=on  InputSameDT=on
  Sum4 : Sum  Inputs=-+|  SaturateOnIntegerOverflow=on  InputSameDT=on
  phidr : Integrator  InitialCondition=phirdo
  phiqr : Integrator  InitialCondition=phirqo
  web1 : Gain  Gain=web_psb  SaturateOnIntegerOverflow=on
  web_psb : Gain  Gain=web_psb  SaturateOnIntegerOverflow=on
  iqr,idr : Outport
  phiqr,phidr : Outport  Port=2
  wires:
  Mux3/1 -> phiqr,phidr/1
  phiqr/1 -> Mux3/1, Product1/2, Sum3/1  "phiqr"
  web1/1 -> phidr/1
  Sum1/1 -> web1/1
  w-wr/1 -> Product/2, Product1/1
  Product/1 -> Sum2/2
  web_psb/1 -> phiqr/1
  Sum2/1 -> web_psb/1
  phidr/1 -> Sum4/2, Product/1, Mux3/2
  vqr,vdr/1 -> Demux/1
  Product1/1 -> Sum1/1
  Demux/2 -> Sum1/2
  1\Llr3/1 -> Sum1/3
  1\Llr2/1 -> 1\Llr3/1, Mux2/2  "idr"
  Sum4/1 -> 1\Llr2/1
  Demux1/2 -> Sum4/1
  Mux2/1 -> iqr,idr/1
  1\Llr/1 -> Mux2/1, 1\Llr1/1  "iqr"
  1\Llr1/1 -> Sum2/3
  Sum3/1 -> 1\Llr/1
  Demux/1 -> Sum2/1
  Demux1/1 -> Sum3/2
  phimq,phimd/1 -> Demux1/1

== system powerlib_modelsV2/Continuous/asynchronous_machine/Stator ==
  phimq,phimd : Inport  Port=1  LatchInput=off
  vqs,vds : Inport  Port=2  LatchInput=off
  w : Inport  Port=3  LatchInput=off
  1\Llr : Gain  Gain=1/Lls  SaturateOnIntegerOverflow=on
  1\Llr1 : Gain  Gain=Rs  SaturateOnIntegerOverflow=on
  1\Llr2 : Gain  Gain=1/Lls  SaturateOnIntegerOverflow=on
  1\Llr3 : Gain  Gain=Rs  SaturateOnIntegerOverflow=on
  Demux : Demux  Outputs=2
  Demux1 : Demux  Outputs=2
  Mux2 : Mux  Inputs=2
  Mux3 : Mux  Inputs=2
  Mux4 : Mux  Inputs=2
  Product : Product  SaturateOnIntegerOverflow=on  InputSameDT=on
  Product1 : Product  SaturateOnIntegerOverflow=on  InputSameDT=on
  Sum1 : Sum  Inputs=++-||  SaturateOnIntegerOverflow=on  InputSameDT=on
  Sum2 : Sum  Inputs=--+  SaturateOnIntegerOverflow=on  InputSameDT=on
  Sum3 : Sum  Inputs=-+  SaturateOnIntegerOverflow=on  InputSameDT=on
  Sum4 : Sum  Inputs=+-|  SaturateOnIntegerOverflow=on  InputSameDT=on
  phids : Integrator  InitialCondition=phisdo
  phiqs : Integrator  InitialCondition=phisqo
  web1 : Gain  Gain=web_psb  SaturateOnIntegerOverflow=on
  web_psb : Gain  Gain=web_psb  SaturateOnIntegerOverflow=on
  phiqs,phids : Outport
  iqs,ids : Outport  Port=2
  phis,is : Outport  Port=3
  wires:
  phimq,phimd/1 -> Demux1/1
  Demux1/1 -> Sum4/2
  Sum4/1 -> 1\Llr/1
  1\Llr/1 -> Mux2/1, 1\Llr1/1  "iqs"
  1\Llr1/1 -> Sum2/1
  vqs,vds/1 -> Demux/1
  Sum2/1 -> web_psb/1
  Demux/1 -> Sum2/3
  Product/1 -> Sum2/2
  web_psb/1 -> phiqs/1
  phiqs/1 -> Mux3/1, Product1/2, Sum4/1
  Mux2/1 -> iqs,ids/1, Mux4/2
  w/1 -> Product/1, Product1/1
  Demux1/2 -> Sum3/1
  Sum3/1 -> 1\Llr2/1
  1\Llr2/1 -> 1\Llr3/1, Mux2/2  "ids"
  1\Llr3/1 -> Sum1/3
  web1/1 -> phids/1
  Sum1/1 -> web1/1
  phids/1 -> Product/2, Sum3/2, Mux3/2
  Demux/2 -> Sum1/2
  Product1/1 -> Sum1/1
  Mux3/1 -> phiqs,phids/1, Mux4/1
  Mux4/1 -> phis,is/1

== system powerlib_modelsV2/Continuous/asynchronous_machine/abc2qd ==
  v : Inport  Port=1  LatchInput=off
  sin,cos : Inport  Port=2  LatchInput=off
  1_Vb : Gain  Gain=1/Vb  SaturateOnIntegerOverflow=on
  Constant : Constant  Orientation=down  Value=ctrl==1
  Constant1 : Constant  Orientation=down  Value=ctrl==2
  Constant2 : Constant  Orientation=down  Value=ctrl==3
  Constant3 : Constant  Orientation=down  Value=ctrl
  Constant4 : Constant  Orientation=left  Value=ctrl
  Multiport Switch : MultiPortSwitch  Inputs=3  InputSameDT=on
  Multiport Switch1 : MultiPortSwitch  Inputs=3  InputSameDT=on
  Mux : Mux  Inputs=2
  Rotor reference frame : Subsystem  TreatAsAtomicUnit=on
      mask Display: disp('Rotor\nreference\nframe')
  Stationary reference frame : Subsystem  TreatAsAtomicUnit=on
      mask Display: disp('Stationary\nreference\nframe')
  Synchronous reference frame : Subsystem  TreatAsAtomicUnit=on
      mask Display: disp('Synchronous\nreference\nframe')
  transit : Subsystem
  vqr,vdr : Outport
  vqs,vds : Outport  Port=2
  wires:
  transit/1(vr,vs) -> 1_Vb/1
  Constant4/1 -> Multiport Switch1/1
  Constant3/1 -> Multiport Switch/1
  1_Vb/1 -> Mux/1
  Mux/1 -> Synchronous reference frame/1(In1), Stationary reference frame/1(In1), Rotor reference frame/1(In1)
  sin,cos/1 -> Mux/2
  Multiport Switch/1 -> vqr,vdr/1
  Synchronous reference frame/2(vqs,vds) -> Multiport Switch1/4
  Stationary reference frame/2(vqs,vds) -> Multiport Switch1/3
  Rotor reference frame/2(vqs,vds) -> Multiport Switch1/2
  Synchronous reference frame/1(vqr,vdr) -> Multiport Switch/4
  Stationary reference frame/1(vqr,vdr) -> Multiport Switch/3
  Rotor reference frame/1(vqr,vdr) -> Multiport Switch/2
  Multiport Switch1/1 -> vqs,vds/1
  Constant2/1 -> Synchronous reference frame/Enable
  Constant1/1 -> Stationary reference frame/Enable
  Constant/1 -> Rotor reference frame/Enable
  v/1 -> transit/1(vu)

== system powerlib_modelsV2/Continuous/asynchronous_machine/dq2abc ==
  sin,cos : Inport  Port=1  LatchInput=off
  iqr,idr : Inport  Port=2  LatchInput=off
  iqs,ids : Inport  Port=3  LatchInput=off
  Constant : Constant  Orientation=down  Value=ctrl==1
  Constant1 : Constant  Orientation=down  Value=ctrl==2
  Constant2 : Constant  Orientation=down  Value=ctrl==3
  Constant3 : Constant  Orientation=down  Value=ctrl
  Constant4 : Constant  Orientation=left  Value=ctrl
  Multiport Switch : MultiPortSwitch  Inputs=3  InputSameDT=on
  Multiport Switch1 : MultiPortSwitch  Inputs=3  InputSameDT=on
  Mux : Mux  Inputs=3
  Mux1 : Mux  Inputs=2
  Mux2 : Mux  Inputs=2
  Mux3 : Mux  Inputs=2
  Rotor reference frame : Subsystem  TreatAsAtomicUnit=on
      mask Display: disp('Rotor\nreference\nframe')
  Selector : Selector  Elements=elements2  InputPortWidth=4
  Stationary reference frame : Subsystem  TreatAsAtomicUnit=on
      mask Display: disp('Stationary\nreference\nframe')
  Sum2 : Sum  Inputs=-  SaturateOnIntegerOverflow=on  InputSameDT=on
  Sum3 : Sum  Inputs=-  SaturateOnIntegerOverflow=on  InputSameDT=on
  Synchronous reference frame : Subsystem  TreatAsAtomicUnit=on
      mask Display: disp('Synchronous\nreference\nframe')
  ib : Gain  Gain=ib  SaturateOnIntegerOverflow=on
  irab,isab : Outport
  irabc : Outport  Port=2
  isabc : Outport  Port=3
  wires:
  Selector/1 -> irab,isab/1
  ib/1 -> Selector/1
  Mux3/1 -> isabc/1
  Sum3/1 -> Mux3/2
  Constant4/1 -> Multiport Switch1/1
  Constant3/1 -> Multiport Switch/1
  Mux1/1 -> ib/1
  Rotor reference frame/2(isa,isb) -> Multiport Switch1/2
  sin,cos/1 -> Mux/3
  Sum2/1 -> Mux2/2
  Multiport Switch1/1 -> Mux3/1, Sum3/1, Mux1/2
  Mux2/1 -> irabc/1
  Multiport Switch/1 -> Sum2/1, Mux1/1, Mux2/1
  iqr,idr/1 -> Mux/1
  iqs,ids/1 -> Mux/2
  Mux/1 -> Synchronous reference frame/1(In1), Stationary reference frame/1(In1), Rotor reference frame/1(In1)
  Synchronous reference frame/2(isa,isb) -> Multiport Switch1/4
  Stationary reference frame/2(isa,isb) -> Multiport Switch1/3
  Synchronous reference frame/1(ira,irb) -> Multiport Switch/4
  Stationary reference frame/1(ira,irb) -> Multiport Switch/3
  Rotor reference frame/1(ira,irb) -> Multiport Switch/2
  Constant2/1 -> Synchronous reference frame/Enable
  Constant1/1 -> Stationary reference frame/Enable
  Constant/1 -> Rotor reference frame/Enable

== system powerlib_modelsV2/Continuous/asynchronous_machine/sin,cos ==
  thr,wr : Inport  Port=1  LatchInput=off
  Constant : Constant  Orientation=down  Value=ctrl<3
  Constant1 : Constant  Value=ctrl
  Constant2 : Constant  Value=0
  Constant3 : Constant  Orientation=down  Value=ctrl==3
  Constant4 : Constant  Value=ctrl
  Constant5 : Constant  Value=0
  Constant6 : Constant
  Gain : Gain  Gain=-1  SaturateOnIntegerOverflow=on
  Multiport Switch : MultiPortSwitch  Inputs=3  InputSameDT=on
  Multiport Switch1 : MultiPortSwitch  Inputs=3  InputSameDT=on
  Selector : Selector  InputPortWidth=2
  Selector1 : Selector  Elements=2  InputPortWidth=2
  Switch : Switch  Threshold=0.5  InputSameDT=on
  sin(beta),cos(beta),sin(th),cos(th) : Subsystem  TreatAsAtomicUnit=on
  sin(thr),cos(thr) : Subsystem  TreatAsAtomicUnit=on
  sin,cos : Outport
  w-wr : Outport  Port=2
  w : Outport  Port=3
  wires:
  Constant/1 -> sin(thr),cos(thr)/Enable, Switch/2
  thr,wr/1 -> Selector/1, sin(beta),cos(beta),sin(th),cos(th)/1(thr,wr), Selector1/1
  Selector/1 -> sin(thr),cos(thr)/1(thr)
  Switch/1 -> sin,cos/1
  Constant3/1 -> sin(beta),cos(beta),sin(th),cos(th)/Enable
  sin(beta),cos(beta),sin(th),cos(th)/2(we-wr) -> Multiport Switch/4
  Constant1/1 -> Multiport Switch/1
  Constant2/1 -> Multiport Switch/2
  Multiport Switch/1 -> w-wr/1
  sin(thr),cos(thr)/1(sin(thr),cos(thr)) -> Switch/1
  sin(beta),cos(beta),sin(th),cos(th)/1("sin(beta),cos(beta), sin(th),cos(th)") -> Switch/3
  Gain/1 -> Multiport Switch/3  "-wr"
  Selector1/1 -> Gain/1, Multiport Switch1/2
  Constant4/1 -> Multiport Switch1/1
  Constant5/1 -> Multiport Switch1/3
  Constant6/1 -> Multiport Switch1/4
  Multiport Switch1/1 -> w/1

== system powerlib_modelsV2/Continuous/breaker/Break Algebraic Loop ==
  In1 : Inport  Port=1  LatchInput=off
  0 2 : Constant  Value=0.001
  Data Type  Conversion : DataTypeConversion  SaturateOnIntegerOverflow=on  RndMeth=Zero
  Data Type  Conversion1 : DataTypeConversion  SaturateOnIntegerOverflow=on  RndMeth=Zero
  Integrator : Integrator  InitialCondition=0.00101*(istate&1)  LimitOutput=on  UpperSaturationLimit=0.00101
  R_device : Gain  Gain=1e7  SaturateOnIntegerOverflow=on
  Relational Operator1 : RelationalOperator  Operator=>  InputSameDT=on
  Vak-Vf-Ron*Iak : Sum  Inputs=+-  SaturateOnIntegerOverflow=on  InputSameDT=on
  Out1 : Outport
  wires:
  Data Type  Conversion/1 -> Out1/1
  In1/1 -> Data Type  Conversion1/1
  Data Type  Conversion1/1 -> Vak-Vf-Ron*Iak/1
  R_device/1 -> Integrator/1
  Vak-Vf-Ron*Iak/1 -> R_device/1
  Integrator/1 -> Vak-Vf-Ron*Iak/2, Relational Operator1/1
  0 2/1 -> Relational Operator1/2
  Relational Operator1/1 -> Data Type  Conversion/1

== system powerlib_modelsV2/Continuous/detailed_thyristor (logical)/Break Alg. Loop ==
  In1 : Inport  Port=1  LatchInput=off
  0 2 : Constant  Value=0.001
  Data Type  Conversion : DataTypeConversion  SaturateOnIntegerOverflow=on  RndMeth=Zero
  Data Type  Conversion1 : DataTypeConversion  SaturateOnIntegerOverflow=on  RndMeth=Zero
  Integrator : Integrator  LimitOutput=on  UpperSaturationLimit=0.00101
  R_device : Gain  Gain=1e7  SaturateOnIntegerOverflow=on
  Relational Operator1 : RelationalOperator  Operator=>  InputSameDT=on
  Vak-Vf-Ron*Iak : Sum  Inputs=+-  SaturateOnIntegerOverflow=on  InputSameDT=on
  Out1 : Outport
  wires:
  Relational Operator1/1 -> Data Type  Conversion/1
  0 2/1 -> Relational Operator1/2
  Integrator/1 -> Relational Operator1/1, Vak-Vf-Ron*Iak/2
  Vak-Vf-Ron*Iak/1 -> R_device/1
  R_device/1 -> Integrator/1
  Data Type  Conversion1/1 -> Vak-Vf-Ron*Iak/1
  In1/1 -> Data Type  Conversion1/1
  Data Type  Conversion/1 -> Out1/1

== system powerlib_modelsV2/Continuous/diode (logical)/Break Alg. Loop ==
  In1 : Inport  Port=1  LatchInput=off
  0 2 : Constant  Value=0.001
  Data Type  Conversion : DataTypeConversion  SaturateOnIntegerOverflow=on  RndMeth=Zero
  Data Type  Conversion1 : DataTypeConversion  SaturateOnIntegerOverflow=on  RndMeth=Zero
  Integrator : Integrator  LimitOutput=on  UpperSaturationLimit=0.00101
  R_device : Gain  Gain=1e7  SaturateOnIntegerOverflow=on
  Relational Operator1 : RelationalOperator  Operator=>  InputSameDT=on
  Vak-Vf-Ron*Iak : Sum  Inputs=+-  SaturateOnIntegerOverflow=on  InputSameDT=on
  Out1 : Outport
  wires:
  Relational Operator1/1 -> Data Type  Conversion/1
  0 2/1 -> Relational Operator1/2
  Integrator/1 -> Relational Operator1/1, Vak-Vf-Ron*Iak/2
  Vak-Vf-Ron*Iak/1 -> R_device/1
  R_device/1 -> Integrator/1
  Data Type  Conversion1/1 -> Vak-Vf-Ron*Iak/1
  In1/1 -> Data Type  Conversion1/1
  Data Type  Conversion/1 -> Out1/1

== system powerlib_modelsV2/Continuous/hysteresis_transformer/Hysteresis ( always SI ) ==
  In1 : Inport  Port=1  LatchInput=off
  Hysteresis main loop + Saturation (Lower Part) : Lookup  DialogController=Simulink.DDGSource  InputValues=LowerFlux  OutputValues=Current  SaturateOnIntegerOverflow=on
  Hysteresis main loop + Saturation. (Upper Part) : Lookup  DialogController=Simulink.DDGSource  InputValues=UpperFlux  OutputValues=Current  SaturateOnIntegerOverflow=on
  Memory : Memory
  SI conversion2 : Gain  Gain=ib  SaturateOnIntegerOverflow=on
  Selector : Selector  Elements=2  InputPortWidth=2
  Selector1 : Selector  InputPortWidth=2
  Sign : Signum
  Sum : Sum  Inputs=|+-  SaturateOnIntegerOverflow=on  InputSameDT=on
  Switch1 : Switch  InputSameDT=on
  Switch2 : Switch  Threshold=1.5  InputSameDT=on
  Tr : Display
  pu conversion : Gain  Gain=fb  SaturateOnIntegerOverflow=on
  sfun_psbtransfosat : S-Function  FunctionName=sfun_test  Parameters=fluxinit*fb,HT,indice,-1,Tolerances,initialslope
  Out1 : Outport
  wires:
  Sum/1 -> Sign/1
  SI conversion2/1 -> Switch2/1  "Boucles internes"
  Selector1/1 -> SI conversion2/1
  Selector/1 -> Tr/1, Switch2/2  "Tr"
  Switch1/1 -> Switch2/3
  Switch2/1 -> Out1/1
  sfun_psbtransfosat/1 -> Selector1/1, Selector/1
  pu conversion/1 -> sfun_psbtransfosat/1
  Sign/1 -> Switch1/2  "sens du flux"
  Memory/1 -> Sum/2  "precedent"
  Hysteresis main loop + Saturation. (Upper Part)/1 -> Switch1/3  "courbe principale + Saturation, partie superieure, le flux est en descente, donc sens negatif"
  In1/1 -> pu conversion/1, Hysteresis main loop + Saturation. (Upper Part)/1, Sum/1, Memory/1, Hysteresis main loop + Saturation (Lower Part)/1
  Hysteresis main loop + Saturation (Lower Part)/1 -> Switch1/1  "courbe principale + Saturation, partie du bas, le flux est en monte, donc sens positif"
